simulink model "bubbles"  (R2017b)
settings: Solver=FixedStepDiscrete  StartTime=0.0  StopTime=inf  FixedStep=1/50  RelTol=1e-3  EnableMultiTasking=on
libraries: embdlinuxlib x1
settings Model: SimulationMode=external  Creator=Josef  LastModifiedBy=Josef
settings SolverCC: PositivePriorityOrder=on
settings OptimizationCC: PassReuseOutputArgsThreshold=0  MaxStackSize=64
settings DebuggingCC: ParameterTunabilityLossMsg=error
settings HardwareCC: ProdBitPerPointer=32  ProdBitPerSizeT=32  ProdBitPerPtrDiffT=32  ProdLargestAtomicInteger=Long  ProdLargestAtomicFloat=Double  ProdWordSize=32  ProdHWDeviceType=ARM Compatible->ARM Cortex  UseEmbeddedCoderFeatures=off
settings SFSimCC: MATLABDynamicMemAlloc=off
settings RTWCC: SystemTargetFile=ert.tlc  HardwareBoard=Raspberry Pi  TemplateMakefile=ert_default_tmf  GenerateReport=on  Toolchain=GNU GCC Raspberry Pi  BuildConfiguration=Debug  TargetLang=C++
settings CodeAppCC: ForceParamTrailComments=on  OperatorAnnotations=on
settings ERTTargetCC: TargetLangStandard=C++03 (ISO)  ERTCustomFileBanners=off  SupportContinuousTime=on  SupportNonInlinedSFcns=on  RemoveResetFunc=off  SupportVariableSizeSignals=on  ModelStepFunctionPrototypeControlCompliant=off

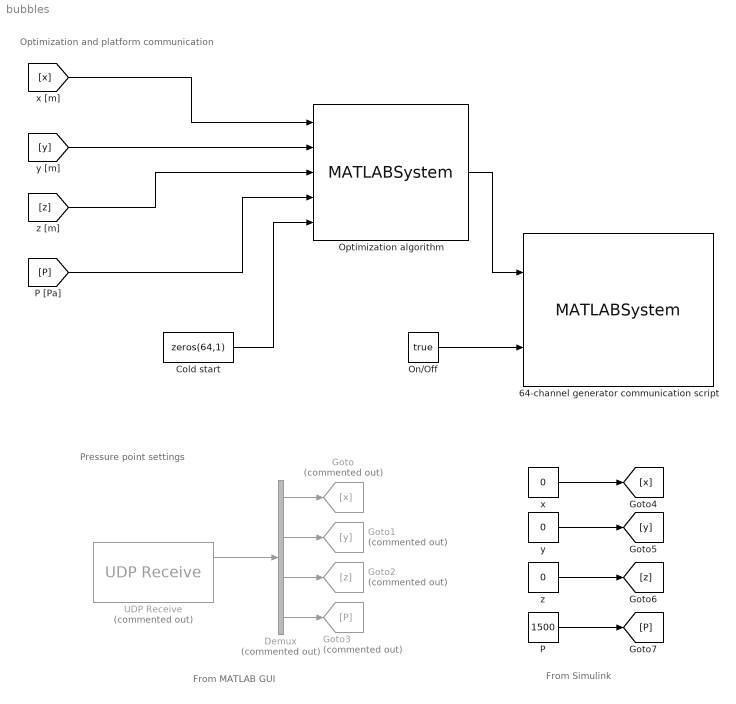
== system bubbles ==
  note: From Simulink
  note: From MATLAB GUI
  note: Pressure point settings
  note: Optimization and platform communication
  64-channel generator communication script : MATLABSystem  System=NewGenerator  Port=/dev/ttyUSB0  Baud=230400
      mask Type: NewGenerator
      mask Display:
      | disp(['64 phase generator' char(10) ' Port: /dev/ttyUSB0' char(10) ' Baudrate: 230400']);
      | port_label('input',1,'phases');
      | port_label('input',2,'On/Off');
  Cold start : Constant  Value=zeros(64,1)
  Demux : Demux  Commented=on
  Goto : Goto  Commented=on  GotoTag=x
  Goto1 : Goto  Commented=on  GotoTag=y
  Goto2 : Goto  Commented=on  GotoTag=z
  Goto3 : Goto  Commented=on  GotoTag=P
  On/Off : Constant  Value=true
  Optimization algorithm : MATLABSystem  System=PressurePoints
      mask Type: PressurePoints
      mask Display:
      | disp(['Pressure points' char(10) 'optimization']);
      | port_label('input',1,'x');
      | port_label('input',2,'y');
      | port_label('input',3,'z');
      | port_label('input',4,'Required pressure');
      | port_label('input',5,'Initial condition');
      | port_label('output',1,'Phases');
  P : Constant  Value=1500
  UDP Receive : embdlinuxlib/UDP Receive  Commented=on  localURL='0.0.0.0'  localPort=25000  remoteURL='0.0.0.0'  remotePort=-1  recvBufferSize=8192  signalDatatype=double  dims=4  isVarSize=off  showBlockingTime=off  blockingTime=0  sampletime=1/50  blockPlatform=Raspberry Pi
      settings: SourceProductName=Simulink Support Package for Raspberry Pi Hardware  SourceProductBaseCode=RASPPI
  x : Constant  Value=0
  y : Constant  Value=0
  z : Constant  Value=0
  wires:
  Optimization algorithm/1 -> 64-channel generator communication script/1
  Cold start/1 -> Optimization algorithm/5
  On/Off/1 -> 64-channel generator communication script/2
  [x] -> Optimization algorithm/1
  [y] -> Optimization algorithm/2
  [P] -> Optimization algorithm/4
  [z] -> Optimization algorithm/3
  Demux/1 -> Goto/1
  UDP Receive/1 -> Demux/1
  Demux/3 -> Goto2/1
  Demux/4 -> Goto3/1
  Demux/2 -> Goto1/1
  P/1 -> [P]
  x/1 -> [x]
  y/1 -> [y]
  z/1 -> [z]
